simulink model "LPV_model_NewBlock"  (R2025b)
settings: Solver=VariableStepAuto  StartTime=0.0  StopTime=200.0  RelTol=1e-3
undefined symbols (not defined in the file or in its folder): M, Na, Nb, NBoccur, Nd, nDelta, nu, nx, ny, str, uss
settings Model: Creator=d.alazard  LastModifiedBy=andre
settings SolverCC: AlgebraicLoopSolver=TrustRegion
settings DebuggingCC: UnconnectedInputMsg=warning  UnconnectedOutputMsg=warning  UnconnectedLineMsg=warning
settings ModelReferenceCC: EnableRefExpFcnMdlSchedulingChecks=on
settings RTWCC: GPUComputeCapability=3.5  DLArmComputeVersion=19.05

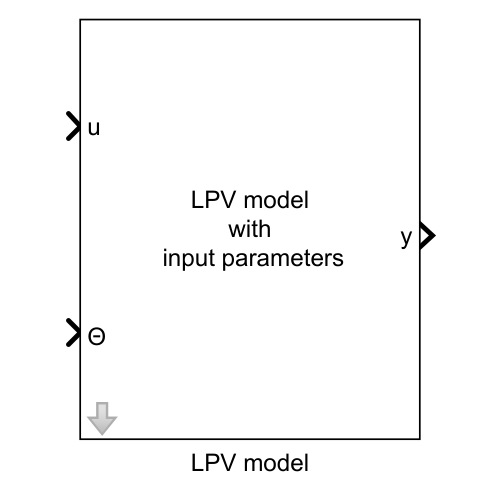
[thumbnail: Simulink's stored preview of the top-level diagram]
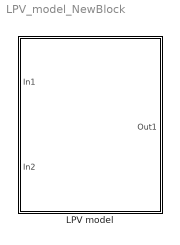
== system LPV_model_NewBlock ==
  LPV model : Subsystem  mask(LPV model with input parameters){Gu=uss(0,1,1,0), RefreshG=Discrete, Tmodel=0.0001, npt=1e-3, TmodelSaved=0.0001, nptSaved=1e-3}
      mask prompts: Gu "Uncertain system (uss)"; RefreshG "Method"; Tmodel "Sampling period (second)"; npt "Normalized parameter variation threshold (>0 and  <1)"; TmodelSaved "Previous sampling period"; nptSaved "previous threshold"
      mask help:
      | This block implements an LPV model (uss generated with the SDTlib).
      | u and y are the classical input and output vectors of the state-space model, noted Gu.
      | \Theta contains the values of the varying parameters (specified as ureal in the uss model).
      | It is assumed that:
      | * the LPV model Gu depends only on real parameters (ureal),
      | * the parameters on the second input of this block are ordered in the same order than the block description of Gu.
      |
      | For faster simulation, it is recommended to update the model in discrete-time. In that case, it is also possible to update the model only when the variation of a normalized parameter (as provided by lfrdata) w.r.t. the previous update is greater that the "normalized parameter varaition threshhold".
      |
      | Note that the "Continuous" and the "Inherit" update methods work only for MATLAB releases R2021a and later. They might require to activate an option: Model settings -> Simulation Target -> Advanced parameters -> Enable continuous-time MATLAB functions to write to initialized persistent variables
      |
      | Made by DYCSYT.
      mask init:
      | init_LPV_model
      mask TypeOptions RefreshG: Inherit | Discrete | Continuous
      mask Callback RefreshG: refreshG_callback
      mask DialogControl Container3 Prompt: Model Update
      mask Display:
      | disp('LPV model\nwith\n input parameters')
      | port_label('input', 1, 'u')
      | port_label('output', 1, 'y')
      | port_label('input',2,'\Theta','interpreter','tex')

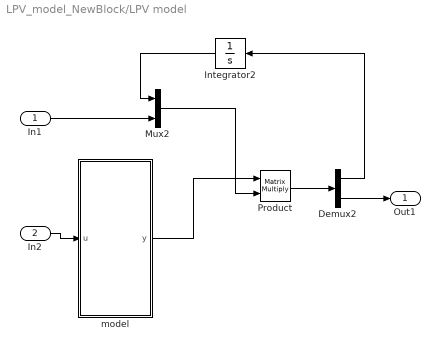
== system LPV_model_NewBlock/LPV model ==
  In1 : Inport
  In2 : Inport  Port=2
  Demux2 : Demux  Outputs=[nx ny]
  Integrator2 : Integrator
  Mux2 : Mux  Inputs=[nx nu]
  Product : Product  Multiplication=Matrix(*)
  model : MATLAB Function  TreatAsAtomicUnit=on  mask{ABCD=[M.a M.b;M.c M.d], nx=nx, nDelta=nDelta, NBoccur=NBoccur, str=str, Na=Na, Nb=Nb, Nd=Nd, npt=npt, yi=zeros(nx+ny,nx+nu), RefreshG=RefreshG}
      mask prompts: ABCD "SS matrics [M.a M.b;M.c M.d] (LFT model)"; nx "number of states nx (integer)"; nDelta "size of the Delta block"; NBoccur "Vecteur of occurrence numbers"; str "Uncertainty structure"; Na "Normalisation parameters Na (vector)"; Nb "Normalisation parameters Nb (vector)"; Nd "Normalisation parameters Nd (vector)"; npt "Normalized parameter variation threshold"; yi "initial value of the y"; RefreshG "Update Method (integer)"
  Out1 : Outport
  wires:
  Demux2/1 -> Integrator2/1
  Integrator2/1 -> Mux2/1
  In1/1 -> Mux2/2
  Product/1 -> Demux2/1
  Mux2/1 -> Product/2
  Demux2/2 -> Out1/1
  model/1(y) -> Product/1
  In2/1 -> model/1(u)

== matlab function LPV_model_NewBlock/LPV model/model ==
  settings: updateMethod=DISCRETE  sampleTime=Tmodel
  data: u input size=Nparam; y output size=[nx+ny,nx+nu]; ABCD parameter; nx parameter; nDelta parameter; NBoccur parameter; str parameter; Na parameter; Nb parameter; Nd parameter; npt parameter; yi parameter; RefreshG parameter
function y   = myfun(u,ABCD,nx,nDelta,NBoccur,str,Na,Nb,Nd,npt,yi,RefreshG)
y=yi;
% Normalization:
u=(Na+Nb.*u)./(1+Nd.*u);
persistent ABCDc p l
if RefreshG==2,
    if isempty(p);
        if length(NBoccur)~=length(u)
            disp('Wrong number of parameter inputs'),
        end
        l=size(ABCD,1);
        p=u;
        delta=u(1)*eye(NBoccur(1));
        for ii=2:length(u),
            delta=blkdiag(delta,u(ii)*eye(NBoccur(ii)));
        end
        ABCDc=[ABCD(:,1:nx) zeros(l,nDelta) ABCD(:,nx+nDelta+1:end)]+...
              ABCD(:,nx+1:nx+nDelta)*inv(eye(nDelta)-delta*ABCD(nx+1:nx+nDelta,nx+1:nx+nDelta))*...
              [delta*ABCD(nx+1:nx+nDelta,1:nx) eye(nDelta) delta*ABCD(nx+1:nx+nDelta,nx+nDelta+1:end)];
    else
        for ii=1:length(u);
            if abs(u(ii)-p(ii))>npt,
                ndii=NBoccur(ii);
                deltaii=(u(ii)-p(ii))*eye(ndii);
                ABCDc=[ABCDc(:,1:str(ii,1)-1) zeros(l,ndii) ABCDc(:,str(ii,2)+1:end)]+...
                ABCDc(:,str(ii,1):str(ii,2))*inv(eye(ndii)-deltaii*ABCDc(str(ii,1):str(ii,2),str(ii,1):str(ii,2)))*...
                [deltaii*ABCDc(str(ii,1):str(ii,2),1:str(ii,1)-1) eye(ndii) deltaii*ABCDc(str(ii,1):str(ii,2),str(ii,2)+1:end)];
                p(ii)=u(ii);
            end
        end
    end
else
    l=size(ABCD,1);
    delta=u(1)*eye(NBoccur(1));
    for ii=2:length(u),
        delta=blkdiag(delta,u(ii)*eye(NBoccur(ii)));
    end
    ABCDc=[ABCD(:,1:nx) zeros(l,nDelta) ABCD(:,nx+nDelta+1:end)]+...
          ABCD(:,nx+1:nx+nDelta)*inv(eye(nDelta)-delta*ABCD(nx+1:nx+nDelta,nx+1:nx+nDelta))*...
          [delta*ABCD(nx+1:nx+nDelta,1:nx) eye(nDelta) delta*ABCD(nx+1:nx+nDelta,nx+nDelta+1:end)];    
end
y(1:end,1:end) = ABCDc([1:nx nx+nDelta+1:end],[1:nx nx+nDelta+1:end]);
end
